simulink model "PMSMCTL"  (R2021a)
settings: Solver=ode23tb  StartTime=0.0  StopTime=1  RelTol=1e-4
values from neighbouring files (symbols this model uses):
  Flux = 0.175    [PMSMCTL_Data.m]
undefined symbols (not defined in the file or in its folder): DiscIntNeverNeededParam
libraries: mcbcontrolslib x3, spsFirstOrderFilterLib x2, simulink x2, eeTransforms x1, spsDCVoltageSourceLib x1, spsPermanentMagnetSynchronousMachineLib x1, spsUniversalBridgeLib x1, spspowerguiLib x1
settings Model: Creator=Administrator  LastModifiedBy=12491
settings SolverCC: AlgebraicLoopSolver=TrustRegion
settings DataIOCC: ReturnWorkspaceOutputs=off
settings DebuggingCC: SFMachineParentedDataDiag=warning  ArithmeticOperatorsInVariantConditions=warning
settings SFSimCC: SimUseLocalCustomCode=off  CustomCodeUndefinedFunction=UseInterfaceOnly
settings RTWCC: RTWUseLocalCustomCode=off

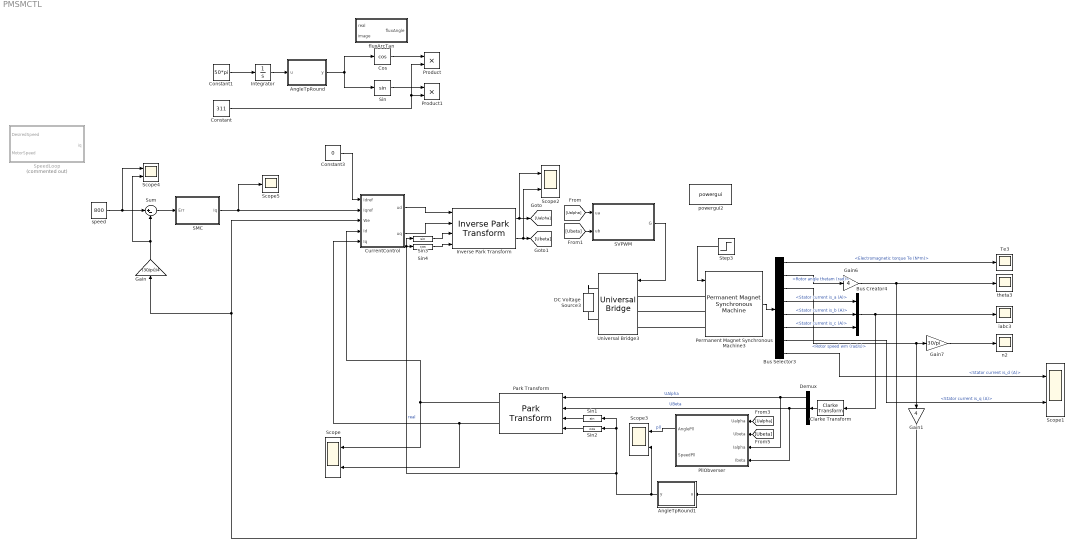
== system PMSMCTL ==
  AngleTpRound : MATLAB Function  TreatAsAtomicUnit=on
  AngleTpRound1 : MATLAB Function  TreatAsAtomicUnit=on
  Bus Creator4 : BusCreator  Inputs=3
  Bus Selector3 : BusSelector  OutputSignals=Electromagnetic torque Te (N*m),Rotor angle thetam (rad),Rotor speed wm (rad/s),Stator current is_a (A),Stator current is_b (A),Stator current is_c (A),Stator current is_q (A),Stator current is_d (A)
  Clarke Transform : eeTransforms/Clarke Transform  PowerInvariant=off
      settings: SourceProductBaseCode=PS
  Constant : Constant  Value=311
  Constant1 : Constant  Value=50*pi
  Constant3 : Constant  Value=0
  Cos : Trigonometry  Operator=cos
  CurrentControl : Subsystem
  DC Voltage Source3 : spsDCVoltageSourceLib/DC Voltage Source  Amplitude=311  Measurements=None
  Demux : Demux  Outputs=3
  Gain : Gain  Gain=(30/pi)/4
  Gain1 : Gain  Gain=4
  Gain6 : Gain  Gain=4
  Gain7 : Gain  Gain=30/pi
  Integrator : Integrator
  Inverse Park Transform : mcbcontrolslib/Inverse Park Transform  AxisAlignment=D-axis
  Park Transform : mcbcontrolslib/Park Transform  AxisAlignment=D-axis
      settings: SourceProductBaseCode=MT
  Permanent Magnet Synchronous Machine3 : spsPermanentMagnetSynchronousMachineLib/Permanent Magnet Synchronous Machine  NbPhases=3  FluxDistribution=Sinusoidal  RotorType=Round  MechanicalLoad=Torque Tm  PresetModel=No  ShowDetailedParameters=on  MeasurementBus=off  Resistance=2.875  Inductance=8.5e-3  dqInductances=[5.25e-3,12e-3]  La=0.0085  MachineConstant=Flux linkage established by magnets (V.s)  Flux=0.175  VoltageCst=126.966  TorqueCst=1.05  Flat=120  Mechanical=[0.003 0.008 4 0]  PolePairs=4  InitialConditions=[0,0, 0,0]  InitialConditions5ph=[0 0 0 0 0 0]  RefAngle=Aligned with phase A axis (original Park)  IterativeDiscreteModel=Trapezoidal non iterative  TsBlock=0.000001  TsPowergui=0
  PllObverser : Subsystem
  Product : Product
  Product1 : Product
  SMC : Subsystem
  SVPWM : Subsystem
  Scope{,1..4} (5 alike) : Scope  NumInputPorts=2
  Scope5 : Scope
  Sin : Trigonometry
  Sin1 : Trigonometry
  Sin2 : Trigonometry  Operator=cos
  Sin3 : Trigonometry
  Sin4 : Trigonometry  Operator=cos
  SpeedLoop : Subsystem  Commented=on
  Step3 : Step  Time=0.5  After=10  SampleTime=0
  Sum : Sum  Inputs=|+-
  Te3 : Scope
  Universal Bridge3 : spsUniversalBridgeLib/Universal Bridge  Arms=3  SnubberResistance=1e5  SnubberCapacitance=inf  Device=MOSFET / Diodes  Ron=1e-3  Lon=0  ForwardVoltages="[  0  0  ]"  ForwardVoltage=0  GTOparameters=[ 10e-6 , 20e-6 ]  IGBTparameters=[ 1e-6 , 2e-6 ]  Measurements=None  Measurements_2=None  converterType=Rectifier
  fluxArcTan : MATLAB Function  TreatAsAtomicUnit=on
  iabc3 : Scope
  n2 : Scope
  powergui2 : spspowerguiLib/powergui  Priority=1  SimulationMode=Continuous  SampleTime=50e-6  frequency=60  Iterations=50  frequencyindice=0  Pbase=100e6  ErrMax=1e-4  UnitsV=kV  UnitsW=MW  buscounter=0  FunctionMessages=off  echomessages=off  EnableUseOfTLC=off  CurrentSourceSwitches=off  DisableSnubberDevices=off  DisableRonSwitches=off  DisableVfSwitches=off  DisplayEquations=off  AutomaticDiscreteSolvers=off  SolverType=Tustin/Backward Euler (TBE)  Interpol=off  ExternalGateDelay=off  methode=off  Ts=100  x0status=blocks  SPID=on  SwTol=0  HookPort=off  NonlinearTolerance=1e-4  nMaxIteration=100  ContinueOnMaxIteration=off  RestoreLinks=warning  ResistiveCurrentMeasurement=off  Frange=[0:2:500]  Ylog=off  Xlog=on  ShowGrid=off  save=off  variable=ZData  structure=0  ZoomFFT=off  StartTime=0.0  cycles=1  DisplayStyle=1  fundamental=60  FreqAxis=off  MaxFrequency=1000  frequencyindicesteady=1  RmsSteady=1  display=off
  speed : Constant  Value=800
  theta3 : Scope
  wires:
  Bus Selector3/3 -> Gain1/1, Gain7/1  "<Rotor speed wm (rad/s)>"
  Permanent Magnet Synchronous Machine3/1 -> Bus Selector3/1
  Bus Selector3/4 -> Bus Creator4/1  "<Stator current is_a (A)>"
  Bus Selector3/6 -> Bus Creator4/3  "<Stator current is_c (A)>"
  Gain6/1 -> theta3/1, AngleTpRound1/1(u)
  Bus Selector3/1 -> Te3/1  "<Electromagnetic torque Te (N*m)>"
  Step3/1 -> Permanent Magnet Synchronous Machine3/1
  Bus Selector3/5 -> Bus Creator4/2  "<Stator current is_b (A)>"
  Bus Selector3/2 -> Gain6/1  "<Rotor angle thetam (rad)>"
  Gain7/1 -> n2/1
  SVPWM/1(G) -> Universal Bridge3/1
  Constant/1 -> Product/2, Product1/2
  Constant1/1 -> Integrator/1
  Integrator/1 -> AngleTpRound/1(u)
  Cos/1 -> Product/1
  Sin/1 -> Product1/1
  Bus Creator4/1 -> Clarke Transform/1, iabc3/1
  Demux/1 -> Park Transform/1, PllObverser/3(Ialpha)  "UAlpha"
  Demux/2 -> Park Transform/2, PllObverser/4(Ibeta)  "UBeta"
  [Ualpha] -> SVPWM/1(ua)
  [Ubeta] -> SVPWM/2(ub)
  AngleTpRound/1(y) -> Sin/1, Cos/1
  Bus Selector3/7 -> Scope1/2  "<Stator current is_q (A)>"
  Bus Selector3/8 -> Scope1/1  "<Stator current is_d (A)>"
  [Ualpha] -> PllObverser/1(Ualpha)
  [Ubeta] -> PllObverser/2(Ubeta)
  Clarke Transform/1 -> Demux/1
  Sin2/1 -> Park Transform/4
  Sin1/1 -> Park Transform/3
  AngleTpRound1/1(y) -> Scope3/2, Sin3/1, Sin4/1, Sin2/1, Sin1/1  "real"
  Park Transform/1 -> Scope/1, CurrentControl/4(Id)
  Park Transform/2 -> Scope/2, CurrentControl/5(Iq)
  Gain1/1 -> CurrentControl/3(We), Gain/1
  Inverse Park Transform/1 -> Scope2/1, [Ualpha]
  Inverse Park Transform/2 -> Scope2/2, [Ubeta]
  SMC/1(Iq) -> Scope5/1, CurrentControl/2(Iqref)
  Constant3/1 -> CurrentControl/1(Idref)
  CurrentControl/1(ud) -> Inverse Park Transform/1
  CurrentControl/2(uq) -> Inverse Park Transform/2
  Sin3/1 -> Inverse Park Transform/3
  Sin4/1 -> Inverse Park Transform/4
  PllObverser/1(AnglePll) -> Scope3/1  "pll"
  speed/1 -> Sum/1, Scope4/1
  Gain/1 -> Scope4/2, Sum/2
  Sum/1 -> SMC/1(Err)
  connections:
  DC Voltage Source3/LConn1 -- Universal Bridge3/RConn2
  Permanent Magnet Synchronous Machine3/LConn2 -- Universal Bridge3/LConn2
  Permanent Magnet Synchronous Machine3/LConn1 -- Universal Bridge3/LConn1
  DC Voltage Source3/RConn1 -- Universal Bridge3/RConn1
  Permanent Magnet Synchronous Machine3/LConn3 -- Universal Bridge3/LConn3

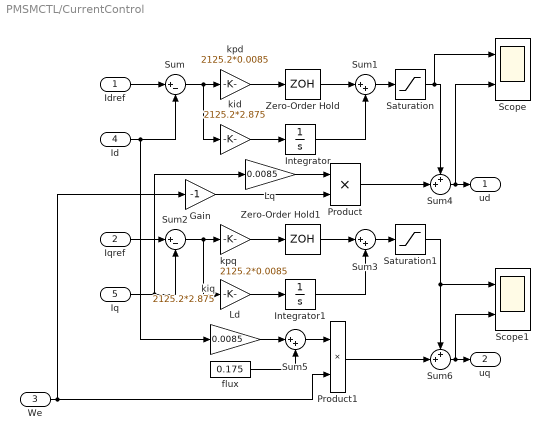
== system PMSMCTL/CurrentControl ==
  Idref : Inport
  Iqref : Inport  Port=2
  We : Inport  Port=3
  Id : Inport  Port=4
  Iq : Inport  Port=5
  Gain : Gain  Gain=-1
  Integrator : Integrator
  Integrator1 : Integrator
  Ld : Gain  Gain=0.0085
  Lq : Gain  Gain=0.0085
  Product : Product
  Product1 : Product
  Saturation : Saturate  UpperLimit=311*0.9*sqrt(1/3)  LowerLimit=-311*0.9*sqrt(1/3)
  Saturation1 : Saturate  UpperLimit=311*0.9*sqrt(1/3)  LowerLimit=-311*0.9*sqrt(1/3)
  Scope : Scope  NumInputPorts=2
  Scope1 : Scope  NumInputPorts=2
  Sum : Sum  Inputs=|+-
  Sum1 : Sum  Inputs=|++
  Sum2 : Sum  Inputs=|+-
  Sum3 : Sum  Inputs=|++
  Sum4 : Sum  Inputs=++|
  Sum5 : Sum  Inputs=|++
  Sum6 : Sum  Inputs=++|
  Zero-Order Hold : ZeroOrderHold  SampleTime=-1
  Zero-Order Hold1 : ZeroOrderHold  SampleTime=-1
  flux : Constant  Value=0.175
  kid : Gain  Gain=2125.2*2.875
  kiq : Gain  Gain=2125.2*2.875
  kpd : Gain  Gain=2125.2*0.0085
  kpq : Gain  Gain=2125.2*0.0085
  ud : Outport
  uq : Outport  Port=2
  wires:
  Idref/1 -> Sum/1
  Id/1 -> Ld/1, Sum/2
  Sum/1 -> kid/1, kpd/1
  kpd/1 -> Zero-Order Hold/1
  kid/1 -> Integrator/1
  Zero-Order Hold/1 -> Sum1/1
  Integrator/1 -> Sum1/2
  Sum1/1 -> Saturation/1
  Saturation/1 -> Scope/1, Sum4/1
  Zero-Order Hold1/1 -> Sum3/1
  Integrator1/1 -> Sum3/2
  Sum3/1 -> Saturation1/1
  kiq/1 -> Integrator1/1
  Iqref/1 -> Sum2/1
  Sum2/1 -> kiq/1, kpq/1
  Saturation1/1 -> Scope1/1, Sum6/1
  kpq/1 -> Zero-Order Hold1/1
  We/1 -> Product1/2, Gain/1
  Iq/1 -> Lq/1, Sum2/2
  Product/1 -> Sum4/2
  Sum4/1 -> Scope/2, ud/1
  Gain/1 -> Product/2
  Lq/1 -> Product/1
  Ld/1 -> Sum5/1
  flux/1 -> Sum5/2
  Sum5/1 -> Product1/1
  Product1/1 -> Sum6/2
  Sum6/1 -> Scope1/2, uq/1

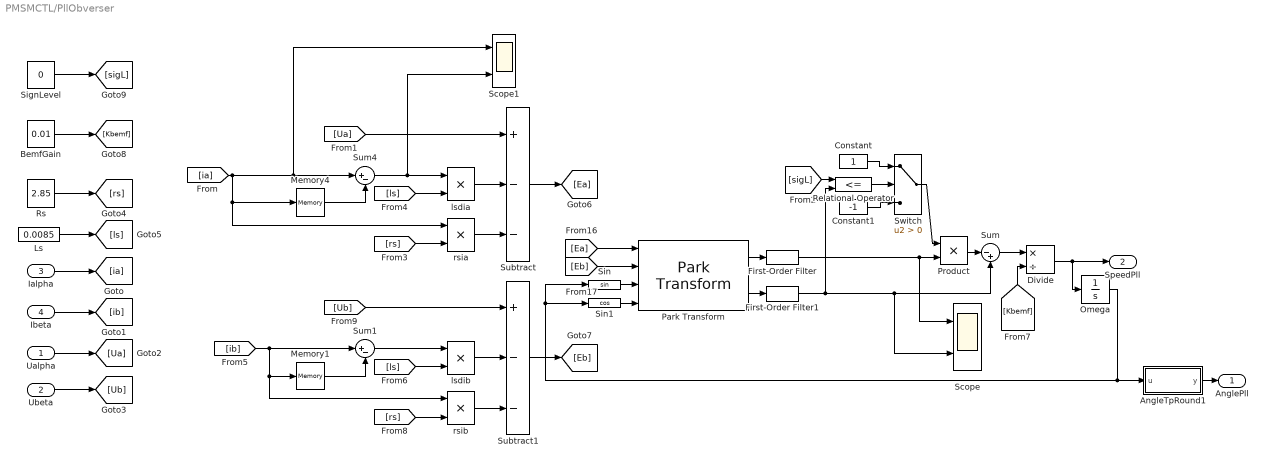
== system PMSMCTL/PllObverser ==
  Ualpha : Inport
  Ubeta : Inport  Port=2
  Ialpha : Inport  Port=3
  Ibeta : Inport  Port=4
  AngleTpRound1 : MATLAB Function  TreatAsAtomicUnit=on
  BemfGain : Constant  Value=0.01
  Constant : Constant
  Constant1 : Constant  Value=-1
  Divide : Product  Inputs=*/
  First-Order Filter : spsFirstOrderFilterLib/First-Order Filter  FilterType=Lowpass  Tc=10e-3  Ts=0  Initialize=on  Vac_Init=[0, 0, 60]  Vdc_Init=0  PlotResponse=off  FreqRange="[0,  200,  1]"
  First-Order Filter1 : spsFirstOrderFilterLib/First-Order Filter  FilterType=Lowpass  Tc=10e-3  Ts=0  Initialize=on  Vac_Init=[0, 0, 60]  Vdc_Init=0  PlotResponse=off  FreqRange="[0,  200,  1]"
  Ls : Constant  Value=0.0085
  Memory1 : Memory  InheritSampleTime=on
  Memory4 : Memory  InheritSampleTime=on
  Omega : Integrator
  Park Transform : mcbcontrolslib/Park Transform  AxisAlignment=D-axis
      settings: SourceProductBaseCode=MT
  Product : Product
  Relational Operator : RelationalOperator  Operator=<=  OutDataTypeStr=boolean  RndMeth=Simplest
  Rs : Constant  Value=2.85
  Scope : Scope  NumInputPorts=2
  Scope1 : Scope  NumInputPorts=2
  SignLevel : Constant  Value=0
  Sin : Trigonometry
  Sin1 : Trigonometry  Operator=cos
  Subtract : Sum  Inputs=+--
  Subtract1 : Sum  Inputs=+--
  Sum : Sum  Inputs=|-+
  Sum1 : Sum  Inputs=|+-
  Sum4 : Sum  Inputs=|+-
  Switch : Switch  Criteria=u2 > Threshold
  lsdia : Product
  lsdib : Product
  rsia : Product
  rsib : Product
  AnglePll : Outport
  SpeedPll : Outport  Port=2
  wires:
  Ialpha/1 -> [ia]
  Ibeta/1 -> [ib]
  Ualpha/1 -> [Ua]
  Ubeta/1 -> [Ub]
  Rs/1 -> [rs]
  Ls/1 -> [ls]
  [ls] -> lsdia/2
  [rs] -> rsia/2
  lsdia/1 -> Subtract/2
  rsia/1 -> Subtract/3
  Subtract/1 -> [Ea]
  Sum1/1 -> lsdib/1
  lsdib/1 -> Subtract1/2
  [ib] -> rsib/1, Memory1/1, Sum1/1
  [rs] -> rsib/2
  [Ub] -> Subtract1/1
  Subtract1/1 -> [Eb]
  rsib/1 -> Subtract1/3
  [ls] -> lsdib/2
  Memory1/1 -> Sum1/2
  Sum4/1 -> Scope1/2, lsdia/1
  Memory4/1 -> Sum4/2
  [Ua] -> Subtract/1
  [ia] -> Scope1/1, Sum4/1, Memory4/1, rsia/1
  [Ea] -> Park Transform/1
  [Eb] -> Park Transform/2
  Omega/1 -> Sin1/1, Sin/1, AngleTpRound1/1(u)
  BemfGain/1 -> [Kbemf]
  Park Transform/1 -> First-Order Filter/1
  Park Transform/2 -> First-Order Filter1/1
  Product/1 -> Sum/1
  Switch/1 -> Product/1
  Constant/1 -> Switch/1
  Constant1/1 -> Switch/3
  Relational Operator/1 -> Switch/2
  SignLevel/1 -> [sigL]
  [sigL] -> Relational Operator/1
  First-Order Filter/1 -> Scope/1, Product/2
  First-Order Filter1/1 -> Scope/2, Sum/2, Relational Operator/2
  AngleTpRound1/1(y) -> AnglePll/1
  Sum/1 -> Divide/1
  Divide/1 -> Omega/1, SpeedPll/1
  [Kbemf] -> Divide/2
  Sin/1 -> Park Transform/3
  Sin1/1 -> Park Transform/4

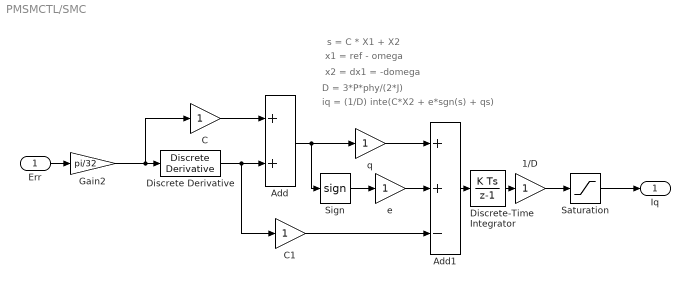
== system PMSMCTL/SMC ==
  note: s = C * X1 + X2
  note: x2 = dx1 = -domega
  note: x1 = ref - omega
  note: D = 3*P*phy/(2*J)
  note: iq = (1/D) inte(C*X2 + e*sgn(s) + qs)
  Err : Inport
  1/D : Gain
  Add : Sum
  Add1 : Sum  Inputs=++-
  C : Gain
  C1 : Gain
  Discrete Derivative : simulink/Discrete/Discrete Derivative  gainval=1.0  ICPrevScaledInput=0.0  OutMin=[]  OutMax=[]  OutDataType=fixdt(1, 16)  OutScaling=2^-10  DoSatur=off
  Discrete-Time Integrator : DiscreteIntegrator  SampleTime=-1  ICPrevOutput=DiscIntNeverNeededParam  ICPrevScaledInput=DiscIntNeverNeededParam
  Gain2 : Gain  Gain=pi/32
  Saturation : Saturate
  Sign : Signum
  e : Gain
  q : Gain
  Iq : Outport
  wires:
  1/D/1 -> Saturation/1
  e/1 -> Add1/2
  Add/1 -> Sign/1, q/1
  Err/1 -> Gain2/1
  Saturation/1 -> Iq/1
  Sign/1 -> e/1
  Discrete Derivative/1 -> C1/1, Add/2
  Gain2/1 -> Discrete Derivative/1, C/1
  C1/1 -> Add1/3
  q/1 -> Add1/1
  Add1/1 -> Discrete-Time Integrator/1
  Discrete-Time Integrator/1 -> 1/D/1
  C/1 -> Add/1

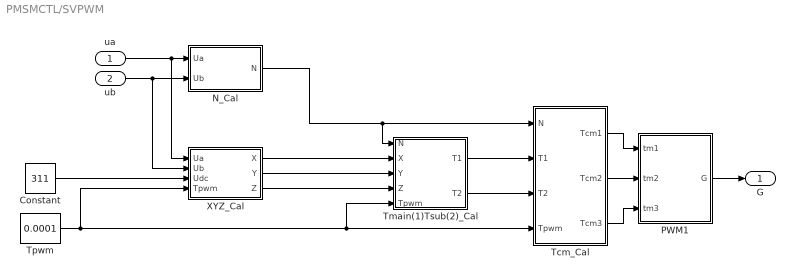
== system PMSMCTL/SVPWM ==
  ua : Inport
  ub : Inport  Port=2
  Constant : Constant  Value=311
  N_Cal : MATLAB Function  TreatAsAtomicUnit=on
  PWM1 : Subsystem
  Tcm_Cal : MATLAB Function  TreatAsAtomicUnit=on
  Tmain(1)Tsub(2)_Cal : MATLAB Function  TreatAsAtomicUnit=on
  Tpwm : Constant  Value=0.0001
  XYZ_Cal : MATLAB Function  TreatAsAtomicUnit=on
  G : Outport  VectorParamsAs1DForOutWhenUnconnected=off
  wires:
  ub/1 -> XYZ_Cal/2(Ub), N_Cal/2(Ub)
  ua/1 -> XYZ_Cal/1(Ua), N_Cal/1(Ua)
  Constant/1 -> XYZ_Cal/3(Udc)
  Tpwm/1 -> XYZ_Cal/4(Tpwm), Tmain(1)Tsub(2)_Cal/5(Tpwm), Tcm_Cal/4(Tpwm)
  Tmain(1)Tsub(2)_Cal/1(T1) -> Tcm_Cal/2(T1)
  Tmain(1)Tsub(2)_Cal/2(T2) -> Tcm_Cal/3(T2)
  XYZ_Cal/3(Z) -> Tmain(1)Tsub(2)_Cal/4(Z)
  N_Cal/1(N) -> Tmain(1)Tsub(2)_Cal/1(N), Tcm_Cal/1(N)
  XYZ_Cal/1(X) -> Tmain(1)Tsub(2)_Cal/2(X)
  XYZ_Cal/2(Y) -> Tmain(1)Tsub(2)_Cal/3(Y)
  Tcm_Cal/2(Tcm2) -> PWM1/2(tm2)
  Tcm_Cal/1(Tcm1) -> PWM1/1(tm1)
  Tcm_Cal/3(Tcm3) -> PWM1/3(tm3)
  PWM1/1(G) -> G/1

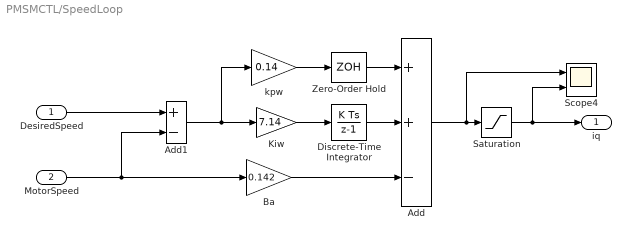
== system PMSMCTL/SpeedLoop ==
  DesiredSpeed : Inport
  MotorSpeed : Inport  Port=2
  Add : Sum  Inputs=++-
  Add1 : Sum  Inputs=+-
  Ba : Gain  Gain=0.142
  Discrete-Time Integrator : DiscreteIntegrator  SampleTime=-1  ICPrevOutput=DiscIntNeverNeededParam  ICPrevScaledInput=DiscIntNeverNeededParam
  Kiw : Gain  Gain=7.14
  Saturation : Saturate  UpperLimit=30  LowerLimit=-30
  Scope4 : Scope  NumInputPorts=2
  Zero-Order Hold : ZeroOrderHold  SampleTime=-1
  kpw : Gain  Gain=0.14
  iq : Outport  VectorParamsAs1DForOutWhenUnconnected=off
  wires:
  Ba/1 -> Add/3
  Saturation/1 -> Scope4/2, iq/1
  kpw/1 -> Zero-Order Hold/1
  Discrete-Time Integrator/1 -> Add/2
  Add/1 -> Scope4/1, Saturation/1
  Kiw/1 -> Discrete-Time Integrator/1
  Zero-Order Hold/1 -> Add/1
  MotorSpeed/1 -> Ba/1, Add1/2
  DesiredSpeed/1 -> Add1/1
  Add1/1 -> kpw/1, Kiw/1

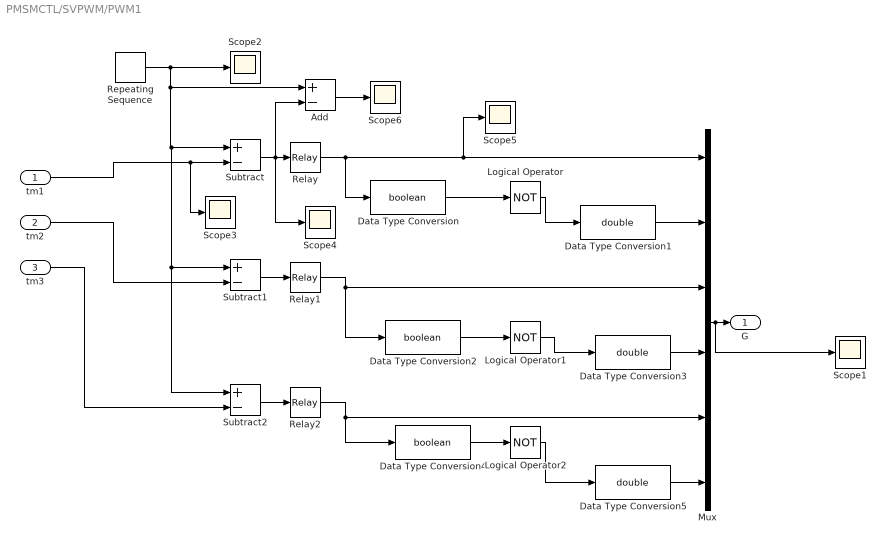
== system PMSMCTL/SVPWM/PWM1 ==
  tm1 : Inport
  tm2 : Inport  Port=2
  tm3 : Inport  Port=3
  Add : Sum  Inputs=+-
  Data Type Conversion : DataTypeConversion  OutDataTypeStr=boolean
  Data Type Conversion1 : DataTypeConversion  OutDataTypeStr=double
  Data Type Conversion2 : DataTypeConversion  OutDataTypeStr=boolean
  Data Type Conversion3 : DataTypeConversion  OutDataTypeStr=double
  Data Type Conversion4 : DataTypeConversion  OutDataTypeStr=boolean
  Data Type Conversion5 : DataTypeConversion  OutDataTypeStr=double
  Logical Operator : Logic  Operator=NOT  AllPortsSameDT=off  OutDataTypeStr=boolean
  Logical Operator1 : Logic  Operator=NOT  AllPortsSameDT=off  OutDataTypeStr=boolean
  Logical Operator2 : Logic  Operator=NOT  AllPortsSameDT=off  OutDataTypeStr=boolean
  Mux : Mux  Inputs=6
  Relay : Relay  ZeroCross=off
  Relay1 : Relay  ZeroCross=off
  Relay2 : Relay  ZeroCross=off
  Repeating Sequence : simulink/Sources/Repeating Sequence  rep_seq_t=[0 0.00005 0.0001]  rep_seq_y=[0 0.0001 0]
  Scope{1..6} (6 alike) : Scope
  Subtract : Sum  Inputs=+-
  Subtract1 : Sum  Inputs=+-
  Subtract2 : Sum  Inputs=+-
  G : Outport  VectorParamsAs1DForOutWhenUnconnected=off
  wires:
  Logical Operator/1 -> Data Type Conversion1/1
  Logical Operator2/1 -> Data Type Conversion5/1
  Logical Operator1/1 -> Data Type Conversion3/1
  tm2/1 -> Subtract1/2
  Relay1/1 -> Data Type Conversion2/1, Mux/3
  tm3/1 -> Subtract2/2
  Relay/1 -> Data Type Conversion/1, Scope5/1, Mux/1
  Relay2/1 -> Data Type Conversion4/1, Mux/5
  Subtract2/1 -> Relay2/1
  Data Type Conversion1/1 -> Mux/2
  tm1/1 -> Scope3/1, Subtract/2
  Subtract1/1 -> Relay1/1
  Data Type Conversion/1 -> Logical Operator/1
  Mux/1 -> Scope1/1, G/1
  Data Type Conversion4/1 -> Logical Operator2/1
  Data Type Conversion5/1 -> Mux/6
  Data Type Conversion2/1 -> Logical Operator1/1
  Data Type Conversion3/1 -> Mux/4
  Repeating Sequence/1 -> Scope2/1, Add/1, Subtract/1, Subtract1/1, Subtract2/1
  Subtract/1 -> Scope4/1, Add/2, Relay/1
  Add/1 -> Scope6/1

== matlab function PMSMCTL/fluxArcTan ==
  data: real input; image input; fluxAngle output
function fluxAngle = fcn(real,image)

    area = 0;
    if(image > 0)
        if(real > 0)
            area = 0;
        else
            area = 1;
        end
    else
        if(real > 0)
            area = 3;
        else
            area = 2;
        end
    end
    
    switch area
        case 0
            fluxAngle = atan(image/real);
        case 1
            fluxAngle = pi + atan(image/real);
        case 2
            fluxAngle = pi + atan(image/real);
        otherwise
            fluxAngle = 2*pi + atan(image/real);
    end

end

== matlab function PMSMCTL/PllObverser/AngleTpRound1 ==
  data: u input; y output
function y = fcn(u)
    factor = u/(2*pi);
    y = 2*pi*(factor - floor(factor));
end

== matlab function PMSMCTL/AngleTpRound ==
  data: u input; y output
function y = fcn(u)
    factor = u/(2*pi);
    y = 2*pi*(factor - floor(factor));
end

== matlab function PMSMCTL/AngleTpRound1 ==
  data: u input; y output
function y = fcn(u)
    factor = u/(2*pi);
    y = 2*pi*(factor - floor(factor));
end

== matlab function PMSMCTL/SVPWM/N_Cal ==
  data: Ua input; N output; Ub input
function N = fcn(Ua, Ub)
    u1 = Ub;
    u2 = sqrt(3)*Ua/2 - Ub/2;
    u3 =-sqrt(3)*Ua/2 - Ub/2;
    
    A = 0;
    B = 0;
    C = 0;
    if u1 > 0
        A = 1;
    end
    
    if u2 > 0
        B = 1;
    end
    
    if u3 > 0
        C = 1;
    end
    

N = 4 * C + 2 * B + A;

== matlab function PMSMCTL/SVPWM/Tcm_Cal ==
  data: N input; Tcm1 output; T1 input; T2 input; Tpwm input; Tcm2 output; Tcm3 output
function [Tcm1, Tcm2, Tcm3] = fcn(N, T1, T2, Tpwm)

    Ta = (Tpwm - T1 - T2)/4;
    Tb = Ta + T1/2;
    Tc = Tb + T2/2;
    
    switch N
        case 1
            Tcm1 = Tb;
            Tcm2 = Ta;
            Tcm3 = Tc;
        case 2
            Tcm1 = Ta;
            Tcm2 = Tc;
            Tcm3 = Tb;
        case 3
            Tcm1 = Ta;
            Tcm2 = Tb;
            Tcm3 = Tc;
        case 4
            Tcm1 = Tc;
            Tcm2 = Tb;
            Tcm3 = Ta;
        case 5
            Tcm1 = Tc;
            Tcm2 = Ta;
            Tcm3 = Tb;
        otherwise
            Tcm1 = Tb;
            Tcm2 = Tc;
            Tcm3 = Ta;
    end

end

== matlab function PMSMCTL/SVPWM/Tmain(1)Tsub(2)_Cal ==
  data: N input; T1 output; X input; Y input; Z input; Tpwm input; T2 output
function [T1, T2] = fcn(N, X, Y, Z, Tpwm)

    switch N
        case 1
            T1 = Z;
            T2 = Y;            
        case 2
            T1 = Y;
            T2 = -X;
        case 3
            T1 = -Z;
            T2 = X;
        case 4 
            T1 = -X;
            T2 = Z;
        case 5
            T1 = X;
            T2 = -Y;
        otherwise
            T1 = -Y;
            T2 = -Z;
    end
    
    if (T1 + T2) > Tpwm
        t1 = T1*Tpwm/(T1+T2);
        t2 = T2*Tpwm/(T1+T2);
        T1 = t1;
        T2 = t2;
    end
end

== matlab function PMSMCTL/SVPWM/XYZ_Cal ==
  data: Ua input; X output; Ub input; Udc input; Tpwm input; Y output; Z output
function [X, Y, Z] = fcn(Ua, Ub, Udc, Tpwm)
    X = sqrt(3)*Tpwm*Ub/Udc;
    Y = Tpwm*(3*Ua/2 + sqrt(3)*Ub/2)/Udc;
    Z = Tpwm*(-3*Ua/2 + sqrt(3)*Ub/2)/Udc;
end
